simulink library "stick_lib"  (R2018b)
settings: Solver=VariableStepAuto  StartTime=0.0  StopTime=10.0  RelTol=1e-3
libraries: $bdroot x1
settings Model: Creator=jonas  LastModifiedBy=jonas

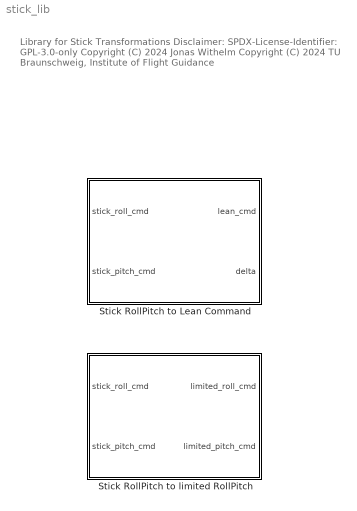
== system stick_lib ==
  note: Library for Stick Transformations
      |
      | Disclaimer:
      | SPDX-License-Identifier: GPL-3.0-only
      |
      | Copyright (C) 2024 Jonas Withelm
      | Copyright (C) 2024 TU Braunschweig, Institute of Flight Guidance
  Stick RollPitch to Lean Command : Subsystem  mask(Stick RollPitch to Lean Command){limiting_mode=int8(1)}
      mask prompts: limiting_mode "Limiting mode (int8):"
      mask help:
      | Converts stick inputs for roll [-1, 1] and pitch [-1, 1] to the lean command "lean_cmd" [0, 1] and "delta" (lean direction).
      |
      | You can choose between two limiting modes that change the scaling behavior of "lean_cmd":
      mask DialogControl TabCircular Prompt: 1: Circular
      mask DialogControl TextCircular Prompt: In circular mode, only a limited value range (of stick inputs) is used. A fixed stick lean angle provides a fixed lean_cmd, independent of the lean direction.
      mask DialogControl TabQuadratic Prompt: 2: Quadratic
      mask DialogControl TextQuadratic Prompt: In quadratic mode, the entire value range (of stick inputs) is used. A fixed stick lean angle provides different values for lean_cmd in dependence of the lean direction.
      mask DialogControl limiting_mode Tooltip: 1: circular, 2: rectangular
  Stick RollPitch to limited RollPitch : Subsystem  mask(Stick RollPitch to limited RollPitch){limiting_mode=int8(1)}
      mask prompts: limiting_mode "Limiting mode (int8):"
      mask help:
      | Converts stick inputs for roll [-1, 1] and pitch [-1, 1] to limited roll and pitch commands, so that sqrt(roll^2 + pitch^2) <= 1.
      |
      | You can choose between two limiting modes that change the scaling behavior:
      mask TypeOptions limiting_mode: Stick RollPitch to Lean Command/limiting_mode
      mask DialogControl TabCircular Prompt: 1: Circular
      mask DialogControl TextCircular Prompt: In circular mode, only a limited value range (of stick inputs) is used.
      mask DialogControl TabQuadratic Prompt: 2: Quadratic
      mask DialogControl TextQuadratic Prompt: In quadratic mode, the entire value range (of stick inputs) is used.
      mask DialogControl limiting_mode Tooltip: 1: circular, 2: rectangular

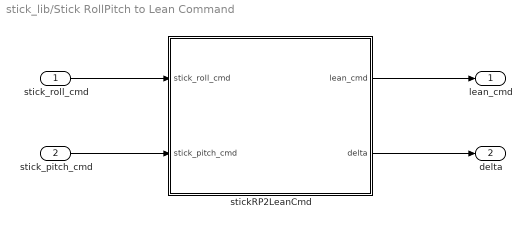
== system stick_lib/Stick RollPitch to Lean Command ==
  stick_roll_cmd : Inport
  stick_pitch_cmd : Inport  Port=2
  stickRP2LeanCmd : MATLAB Function  TreatAsAtomicUnit=on
  lean_cmd : Outport
  delta : Outport  Port=2
  wires:
  stick_roll_cmd/1 -> stickRP2LeanCmd/1(stick_roll_cmd)
  stick_pitch_cmd/1 -> stickRP2LeanCmd/2(stick_pitch_cmd)
  stickRP2LeanCmd/1(lean_cmd) -> lean_cmd/1
  stickRP2LeanCmd/2(delta) -> delta/1

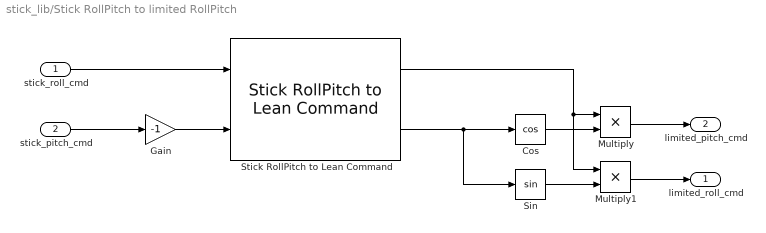
== system stick_lib/Stick RollPitch to limited RollPitch ==
  stick_roll_cmd : Inport
  stick_pitch_cmd : Inport  Port=2
  Cos : Trigonometry  Operator=cos
  Gain : Gain  Gain=-1
  Multiply : Product
  Multiply1 : Product
  Sin : Trigonometry
  Stick RollPitch to Lean Command : $bdroot/Stick RollPitch to Lean Command  limiting_mode=limiting_mode
  limited_roll_cmd : Outport
  limited_pitch_cmd : Outport  Port=2
  wires:
  stick_roll_cmd/1 -> Stick RollPitch to Lean Command/1
  Multiply/1 -> limited_pitch_cmd/1
  Stick RollPitch to Lean Command/1 -> Multiply1/1, Multiply/1
  Multiply1/1 -> limited_roll_cmd/1
  Cos/1 -> Multiply/2
  stick_pitch_cmd/1 -> Gain/1
  Stick RollPitch to Lean Command/2 -> Sin/1, Cos/1
  Sin/1 -> Multiply1/2
  Gain/1 -> Stick RollPitch to Lean Command/2

== matlab function stick_lib/Stick RollPitch to Lean Command/stickRP2LeanCmd ==
  data: stick_roll_cmd input; lean_cmd output; stick_pitch_cmd input; delta output; limiting_mode parameter int8 size=1
function [lean_cmd, delta] = stickRP2LeanCmd(stick_roll_cmd, stick_pitch_cmd, limiting_mode)

[lean_cmd, delta] = stickRP2LeanCmd(stick_roll_cmd, stick_pitch_cmd, limiting_mode);

end
